simulink model "ERP_NF_huji"  (R2015a)
settings: Solver=ode45  SolverMode=SingleTasking  StartTime=0.0  StopTime=Inf  RelTol=1e-3
model workspace (MAT data in the model file):
  device_serial = 'HA-2016.07.01'
  sample_rate = 256
  buffer_size = 1
  number_of_channels = 11
  cfg_native : struct (value not decoded)
undefined symbols (not defined in the file): HA
libraries: gHIampLib x1, gHIampTools x1, gtecHighspeedLib x1
settings Model: CovSFcnEnable=off  Creator=cognitive  LastModifiedBy=Michael
settings OptimizationCC: BlockReduction=off  BooleanDataType=off
settings DebuggingCC: SaveWithParameterizedLinksMsg=none  UnderspecifiedInitializationDetection=Classic  MergeDetectMultiDrivingBlocksExec=none  SignalResolutionControl=TryResolveAllWithWarning
settings HardwareCC: TargetUnknown=on

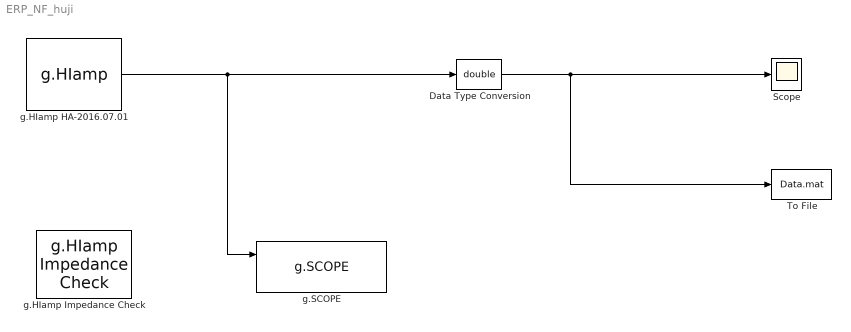
== system ERP_NF_huji ==
  Data Type Conversion : DataTypeConversion  OutDataTypeStr=double
  Scope : Scope
      settings: TimeRange=10  YMin=-40  YMax=30
  To File : ToFile  StartFcn=% cd C:\Users\sareld\Documents\eeg-rl\eeg-rl\experiment\code\matlab  StopFcn=|  Filename=Data.mat  MatrixName=full_data  SaveFormat=Timeseries
      | dataFilename = input('Enter file name for saving the current data','s');
      | dirName = [dataFilename '_' datestr(datetime('today'))];
      | mkdir (['Z:\EEG_Data\Car_Game_NF\' dirName])
      | copyfile('Data.mat',['Z:\EEG_Data\Car_Game_NF\' dirName '\Data_' dataFilename '_' datestr(datetime('today')) '.mat'],'f');
  g.HIamp HA-2016.07.01 : gHIampLib/g.HIamp  sample_rate=256  buffer_size=1  number_of_channels=11  device_serial=HA-2016.07.01
  g.HIamp Impedance Check : gHIampTools/g.HIamp Impedance Check
  g.SCOPE : gtecHighspeedLib/g.SCOPE
  wires:
  g.HIamp HA-2016.07.01/1 -> g.SCOPE/1, Data Type Conversion/1
  Data Type Conversion/1 -> To File/1, Scope/1
